simulink model "c71_car0_template"  (R2025b)
settings: Solver=FixedStepDiscrete  StartTime=0.0  StopTime=inf  FixedStep=P_dt  RelTol=1e-3
InitFcn:
  | rosenv;
  | s06_data;
model workspace (MAT data in the model file):
  SL_ROS_VariableLengthArrays_MaxSizes.CommonInfo.ArrayTruncateAction = 'DoNothing'
  SL_ROS_VariableLengthArrays_MaxSizes.MsgTypeMap = containers.Map
  SL_ROS_VariableLengthArrays_MaxSizes.MsgTypeMap.serialization.keys = {'mbmadmsgs/CarObsList', 'mbmadmsgs/CarOutputsExtList', 'mbmadmsgs/DriveManeuver', 'mbsafemsgs/CheckpointSequence'}
  SL_ROS_VariableLengthArrays_MaxSizes.MsgTypeMap.serialization.values{1}.PropertyName = 'list'
  SL_ROS_VariableLengthArrays_MaxSizes.MsgTypeMap.serialization.values{1}.DataType = 'mbmadmsgs/CarObs'
  SL_ROS_VariableLengthArrays_MaxSizes.MsgTypeMap.serialization.values{1}.MaxLength = 4
  SL_ROS_VariableLengthArrays_MaxSizes.MsgTypeMap.serialization.values{2}.PropertyName = 'list'
  SL_ROS_VariableLengthArrays_MaxSizes.MsgTypeMap.serialization.values{2}.DataType = 'mbmadmsgs/CarOutputsExt'
  SL_ROS_VariableLengthArrays_MaxSizes.MsgTypeMap.serialization.values{2}.MaxLength = 2
  SL_ROS_VariableLengthArrays_MaxSizes.MsgTypeMap.serialization.values{3}(1).PropertyName = 'breaks'
  SL_ROS_VariableLengthArrays_MaxSizes.MsgTypeMap.serialization.values{3}(1).DataType = 'single'
  SL_ROS_VariableLengthArrays_MaxSizes.MsgTypeMap.serialization.values{3}(1).MaxLength = 200
  SL_ROS_VariableLengthArrays_MaxSizes.MsgTypeMap.serialization.values{3}(2).PropertyName = 's1'
  SL_ROS_VariableLengthArrays_MaxSizes.MsgTypeMap.serialization.values{3}(2).DataType = 'single'
  SL_ROS_VariableLengthArrays_MaxSizes.MsgTypeMap.serialization.values{3}(2).MaxLength = 200
  SL_ROS_VariableLengthArrays_MaxSizes.MsgTypeMap.serialization.values{3}(3).PropertyName = 's2'
  SL_ROS_VariableLengthArrays_MaxSizes.MsgTypeMap.serialization.values{3}(3).DataType = 'single'
  SL_ROS_VariableLengthArrays_MaxSizes.MsgTypeMap.serialization.values{3}(3).MaxLength = 200
  SL_ROS_VariableLengthArrays_MaxSizes.MsgTypeMap.serialization.values{3}(4).PropertyName = 'segments'
  SL_ROS_VariableLengthArrays_MaxSizes.MsgTypeMap.serialization.values{3}(4).DataType = 'uint32'
  SL_ROS_VariableLengthArrays_MaxSizes.MsgTypeMap.serialization.values{3}(4).MaxLength = 200
  SL_ROS_VariableLengthArrays_MaxSizes.MsgTypeMap.serialization.values{3}(5).PropertyName = 'spline_coefs1'
  SL_ROS_VariableLengthArrays_MaxSizes.MsgTypeMap.serialization.values{3}(5).DataType = 'single'
  SL_ROS_VariableLengthArrays_MaxSizes.MsgTypeMap.serialization.values{3}(5).MaxLength = 800
  SL_ROS_VariableLengthArrays_MaxSizes.MsgTypeMap.serialization.values{3}(6).PropertyName = 'spline_coefs2'
  SL_ROS_VariableLengthArrays_MaxSizes.MsgTypeMap.serialization.values{3}(6).DataType = 'single'
  SL_ROS_VariableLengthArrays_MaxSizes.MsgTypeMap.serialization.values{3}(6).MaxLength = 800
  SL_ROS_VariableLengthArrays_MaxSizes.MsgTypeMap.serialization.values{4}.PropertyName = 'cpseq'
  SL_ROS_VariableLengthArrays_MaxSizes.MsgTypeMap.serialization.values{4}.DataType = 'mbsafemsgs/Checkpoint'
  SL_ROS_VariableLengthArrays_MaxSizes.MsgTypeMap.serialization.values{4}.MaxLength = 23
  SL_ROS_VariableLengthArrays_MaxSizes.MsgTypeMap.serialization.uniformity = 0
  SL_ROS_VariableLengthArrays_MaxSizes.MsgTypeMap.serialization.keyType = 'char'
  SL_ROS_VariableLengthArrays_MaxSizes.MsgTypeMap.serialization.valueType = 'any'
values from neighbouring files (symbols this model uses):
  P_display_dt = 50e-3    (= 0.05)    [s06_data.m]
  P_dt = 25e-3    (= 0.025)    [s06_data.m]
  P_p_delta_max = 21.58/180*pi    (= 0.37664205258)    [d01_data.m]    (also in d71_data.m = 0.383972435439)
  P_p_deltan_max = 1    [d01_data.m]    (also in d71_data.m = 0.93)
  P_p_deltan_min = -P_p_deltan_max    (= -1)    [d01_data.m]    (also in d71_data.m = -0.93)
  P_p_k = 2.51    [d01_data.m]    (also in d71_data.m = 3.4)
  P_p_l = abs(P_p_frontaxle_1 + P_p_rearaxle_1)    [d01_data.m]    (also in d71_data.m = 0.0325)
  P_p_T = 316e-3    (= 0.316)    [d01_data.m]    (also in d71_data.m = 0.12)
  P_p_Tsteer = 0.3    [d01_data.m]
  P_p_Tt = P_p_uTt + P_p_output_Tt    (= 0.11)    [d01_data.m]    (also in d71_data.m = 0.1)
  P_p_un_max = 1    [d01_data.m]    (also in d71_data.m = 0.2)
  P_p_vRef = 0.2    [baseline_lqr_script.m]    (also in d71_data.m = 0.15)
undefined symbols (not defined in the file or in its folder): carid, CarInputsCmdForward, CarInputsCmdHalt, cmd, cpseq, P_cpseq, P_p_tuneKI, P_p_tuneKP, P_p_un_table, P_p_uref, P_p_vss_table, pedals, steering
libraries: ros2lib x5, mbrt_lib_level1 x2, vrlib x1, eeGeneralControl x1
settings Model: Creator=frank  LastModifiedBy=jty
settings OptimizationCC: EnhancedBackFolding=on  PassReuseOutputArgsAs=Individual arguments  ZeroExternalMemoryAtStartup=off  ZeroInternalMemoryAtStartup=off  MaxStackSize=64  OptimizeBlockOrder=speed  DifferentSizesBufferReuse=on  OptimizationCustomize=off  EfficientTunableParamExpr=on
settings DebuggingCC: ParameterTunabilityLossMsg=error  UnconnectedInputMsg=warning  UnconnectedOutputMsg=warning  UnconnectedLineMsg=warning  BusObjectLabelMismatch=error
settings HardwareCC: ProdBitPerLong=64.0  ProdHWDeviceType=Intel->x86-64 (Linux 64)
settings ModelReferenceCC: EnableRefExpFcnMdlSchedulingChecks=on
settings SFSimCC: MATLABDynamicMemAlloc=off
settings RTWCC: SystemTargetFile=ert.tlc  HardwareBoard=Robot Operating System 2 (ROS 2)  GenCodeOnly=on  TemplateMakefile=ert_default_tmf  GenerateReport=on  Toolchain=Colcon Tools  BuildConfiguration=Faster Runs  IncludeHyperlinkInReport=on  TargetLang=C++  GenerateTraceInfo=on  GPUComputeCapability=3.5  DLArmComputeVersion=19.05  Description=Embedded Coder
settings CodeAppCC: ForceParamTrailComments=on  IgnoreCustomStorageClasses=off  OperatorAnnotations=on  SimulinkDataObjDesc=on  SFDataObjDesc=on  InsertBlockDesc=on
settings ERTTargetCC: ExtModeTransport=2.0  ExtModeStaticAlloc=on  ExtModeAutomaticAllocSize=off  ExtModeMexFile=ext_xcp  ExtModeIntrfLevel=Level2 - Open  InlinedParameterPlacement=Hierarchical  RootIOFormat=Structure reference  DynamicArrayContainerType=coder::array  CodeInterfacePackaging=C++ class  SubcomponentCodeInterfacePackaging=C++ class  SupportNonInlinedSFcns=on  SupportVariableSizeSignals=on

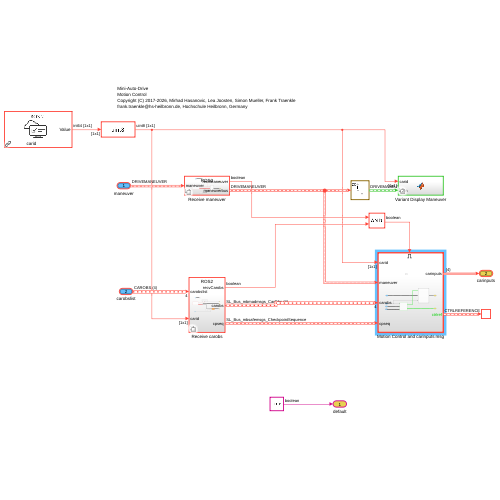
[thumbnail: Simulink's stored preview of the top-level diagram]
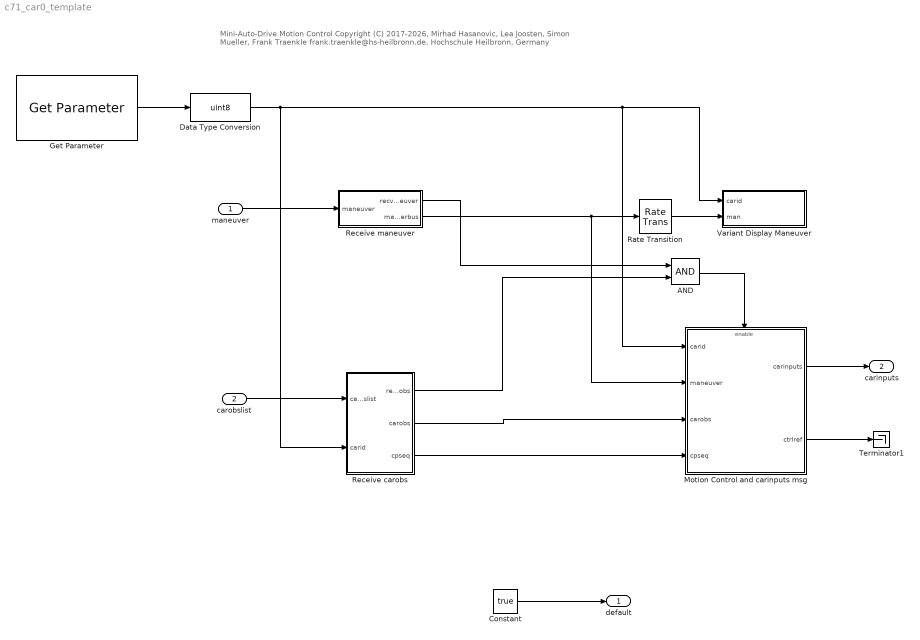
== system c71_car0_template ==
  note: Mini-Auto-Drive
      | Motion Control
      | Copyright (C) 2017-2026, Mirhad Hasanovic, Lea Joosten, Simon Mueller, Frank Traenkle
      | frank.traenkle@hs-heilbronn.de, Hochschule Heilbronn, Germany
  maneuver : Inport  OutDataTypeStr=Bus: DRIVEMANEUVER  BusOutputAsStruct=on
  carobslist : Inport  Port=2  OutDataTypeStr=Bus: CAROBS  PortDimensions=P_car_cnt  BusOutputAsStruct=on
  AND : Logic  AllPortsSameDT=off  OutDataTypeStr=boolean
  Constant : Constant  Value=true
  Data Type Conversion : DataTypeConversion  OutDataTypeStr=uint8  SaturateOnIntegerOverflow=off  RndMeth=Floor
  Get Parameter : ros2lib/Get Parameter  ParameterName=carid  ParameterType=int64  ParameterMaxArrayLength=16  ParameterInitialValue=0  SampleTime=-1  ModelName=c71_car0_template  BlockId=ParamGet_c71_car0_template_2057
  Motion Control and carinputs msg : Subsystem
  Rate Transition : RateTransition
  Receive carobs : Subsystem  Variant=on
  Receive maneuver : Subsystem  Variant=on
  Terminator1 : Terminator
  Variant Display Maneuver : Subsystem  Variant=on  VariantControlMode=sim codegen switching
  default : Outport  BusOutputAsStruct=on
  carinputs : Outport  Port=2  OutDataTypeStr=Bus: CARINPUTS  BusOutputAsStruct=on
  wires:
  Receive maneuver/1(recvManeuver) -> AND/1
  Motion Control and carinputs msg/1(carinputs) -> carinputs/1
  Receive maneuver/2(maneuverbus) -> Motion Control and carinputs msg/2(maneuver), Rate Transition/1
  Motion Control and carinputs msg/2(ctrlref) -> Terminator1/1
  Rate Transition/1 -> Variant Display Maneuver/2(man)
  maneuver/1 -> Receive maneuver/1(maneuver)
  Receive carobs/2(carobs) -> Motion Control and carinputs msg/3(carobs)
  Data Type Conversion/1 -> Receive carobs/2(carid), Motion Control and carinputs msg/1(carid), Variant Display Maneuver/1(carid)
  Receive carobs/3(cpseq) -> Motion Control and carinputs msg/4(cpseq)
  AND/1 -> Motion Control and carinputs msg/Enable
  Receive carobs/1(recvCarobs) -> AND/2
  carobslist/1 -> Receive carobs/1(carobslist)
  Constant/1 -> default/1
  Get Parameter/1 -> Data Type Conversion/1

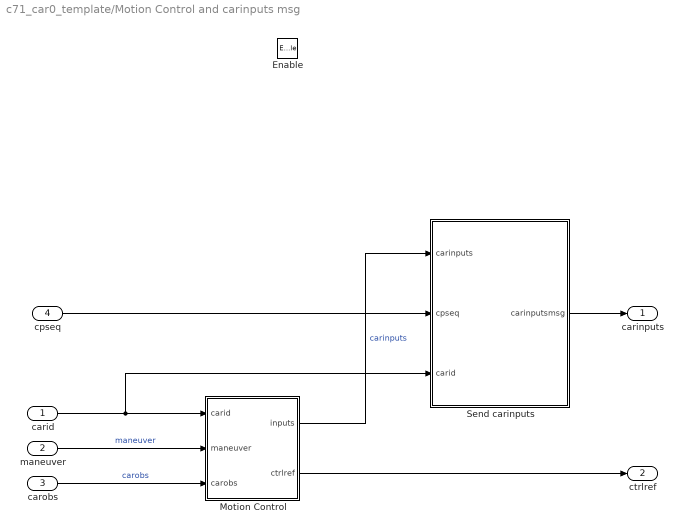
== system c71_car0_template/Motion Control and carinputs msg ==
  carid : Inport
  maneuver : Inport  Port=2
  carobs : Inport  Port=3
  cpseq : Inport  Port=4
  Enable : EnablePort
  Motion Control : Subsystem  TreatAsAtomicUnit=on  SystemSampleTime=P_dt
  Send carinputs : Subsystem  Variant=on
  carinputs : Outport
  ctrlref : Outport  Port=2
  wires:
  Send carinputs/1(carinputsmsg) -> carinputs/1
  carid/1 -> Motion Control/1(carid), Send carinputs/3(carid)
  cpseq/1 -> Send carinputs/2(cpseq)
  Motion Control/1(inputs) -> Send carinputs/1(carinputs)  "carinputs"
  Motion Control/2(ctrlref) -> ctrlref/1
  carobs/1 -> Motion Control/3(carobs)  "carobs"
  maneuver/1 -> Motion Control/2(maneuver)  "maneuver"

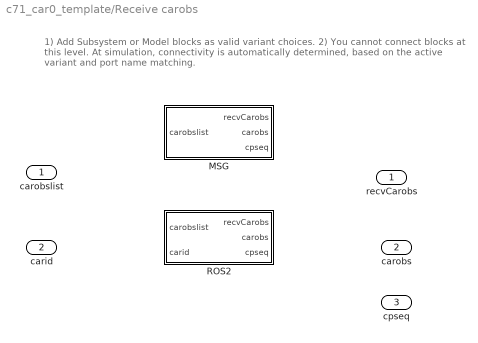
== system c71_car0_template/Receive carobs ==
  note: 1) Add Subsystem or Model blocks as valid variant choices.
      | 2) You cannot connect blocks at this level. At simulation, connectivity is automatically
      | determined, based on the active variant and port name matching.
  carobslist : Inport
  carid : Inport  Port=2
  MSG : Subsystem  VariantControl=VariantCom == VARIANT_COM_TYPE.MSG
  ROS2 : Subsystem  VariantControl=VariantCom == VARIANT_COM_TYPE.ROS2
  recvCarobs : Outport
  carobs : Outport  Port=2
  cpseq : Outport  Port=3

== system c71_car0_template/Receive maneuver ==
  note: 1) Add Subsystem or Model blocks as valid variant choices.
      | 2) You cannot connect blocks at this level. At simulation, connectivity is automatically
      | determined, based on the active variant and port name matching.
  maneuver : Inport
  MSG : Subsystem  VariantControl=VariantCom == VARIANT_COM_TYPE.MSG
  ROS2 : Subsystem  VariantControl=VariantCom == VARIANT_COM_TYPE.ROS2
  recvManeuver : Outport
  maneuverbus : Outport  Port=2

== system c71_car0_template/Variant Display Maneuver ==
  note: 1) Add Subsystem or Model blocks as valid variant choices.
      | 2) You cannot connect blocks at this level. At simulation, connectivity is automatically
      | determined, based on the active variant and port name matching.
  carid : Inport
  man : Inport  Port=2
  DisplayManeuver : MATLAB Function  TreatAsAtomicUnit=on  SystemSampleTime=P_display_dt  VariantControl=(sim)
  None : Subsystem  VariantControl=(codegen)

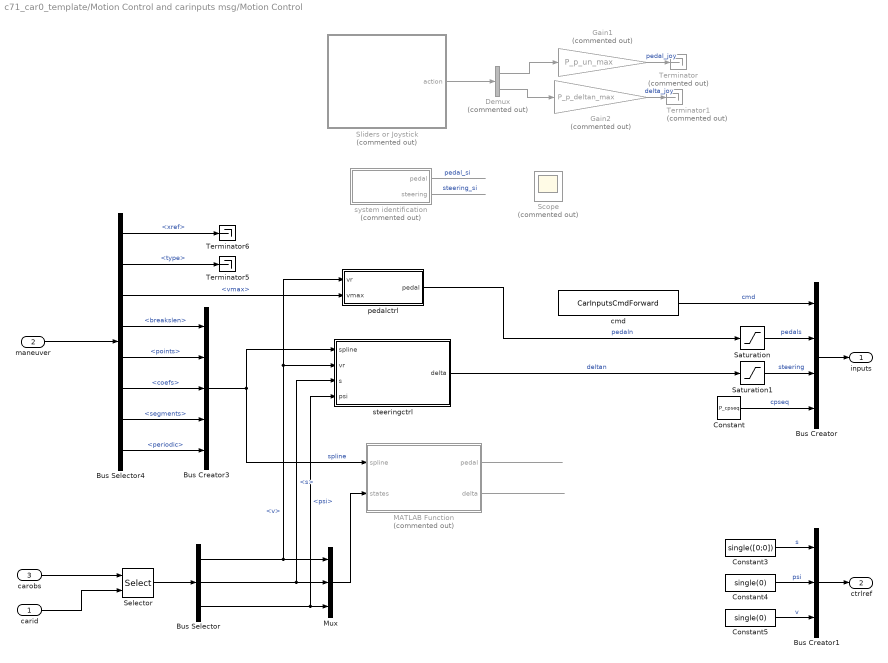
== system c71_car0_template/Motion Control and carinputs msg/Motion Control ==
  carid : Inport
  maneuver : Inport  Port=2
  carobs : Inport  Port=3
  Bus Creator : BusCreator  Inputs=4  OutDataTypeStr=Bus: CARINPUTS  NonVirtualBus=on
  Bus Creator1 : BusCreator  Inputs=3  OutDataTypeStr=Bus: CTRLREFERENCE  NonVirtualBus=on
  Bus Creator3 : BusCreator  Inputs=5  OutDataTypeStr=Bus: SPLINE
  Bus Selector : BusSelector  OutputSignals=v,s,psi
  Bus Selector4 : BusSelector  OutputSignals=xref,type,vmax,breakslen,points,coefs,segments,periodic
  Constant : Constant  Value=P_cpseq  OutDataTypeStr=Bus: CHECKPOINTSEQUENCEMSG
  Constant3 : Constant  Value=single([0;0])
  Constant4 : Constant  Value=single(0)
  Constant5 : Constant  Value=single(0)
  Demux : Demux  Commented=on  Outputs=2
  Gain1 : Gain  Commented=on  Gain=P_p_un_max
  Gain2 : Gain  Commented=on  Gain=P_p_deltan_max
  MATLAB Function : MATLAB Function  Commented=on  TreatAsAtomicUnit=on
  Mux : Mux  Inputs=3
  Saturation : Saturate  UpperLimit=P_p_un_max  LowerLimit=0.03
  Saturation1 : Saturate  UpperLimit=P_p_deltan_max  LowerLimit=P_p_deltan_min
  Scope : Scope  Commented=on  NumInputPorts=2
      settings: ActiveDisplayYMinimum=-0.15337172032176821  ActiveDisplayYMaximum=0.22733787891864379
  Selector : Selector  IndexMode=Zero-based  InputPortWidth=P_car_cnt  IndexOptions=Index vector (port)  Indices=0  OutputSizes=1
  Sliders or Joystick : Subsystem  Commented=on  Variant=on  VariantControlMode=label  LabelModeActiveChoice=true
  Terminator : Terminator  Commented=on
  Terminator1 : Terminator  Commented=on
  Terminator5 : Terminator
  Terminator6 : Terminator
  cmd : Constant  Value=CarInputsCmdForward
  pedalctrl : Subsystem
  steeringctrl : Subsystem
  system identification : Subsystem  Commented=on
  inputs : Outport  VectorParamsAs1DForOutWhenUnconnected=off
  ctrlref : Outport  Port=2  VectorParamsAs1DForOutWhenUnconnected=off
  wires:
  Constant5/1 -> Bus Creator1/3  "v"
  Constant3/1 -> Bus Creator1/1  "s"
  Constant4/1 -> Bus Creator1/2  "psi"
  Bus Creator1/1 -> ctrlref/1
  Constant/1 -> Bus Creator/4  "cpseq"
  Demux/2 -> Gain2/1
  Demux/1 -> Gain1/1
  Sliders or Joystick/1(action) -> Demux/1
  Bus Creator/1 -> inputs/1
  Saturation/1 -> Bus Creator/2  "pedals"
  Saturation1/1 -> Bus Creator/3  "steering"
  cmd/1 -> Bus Creator/1  "cmd"
  Gain2/1 -> Terminator1/1  "delta_joy"
  Gain1/1 -> Terminator/1  "pedal_joy"
  Bus Selector/2 -> steeringctrl/3(s), Mux/2  "<s>"
  carobs/1 -> Selector/1
  Bus Selector/1 -> pedalctrl/1(vr), steeringctrl/2(vr), Mux/1  "<v>"
  Bus Selector/3 -> steeringctrl/4(psi), Mux/3  "<psi>"
  Selector/1 -> Bus Selector/1
  carid/1 -> Selector/2
  Bus Selector4/7 -> Bus Creator3/4  "<segments>"
  Bus Selector4/2 -> Terminator5/1  "<type>"
  maneuver/1 -> Bus Selector4/1
  Bus Selector4/3 -> pedalctrl/2(vmax)  "<vmax>"
  Bus Selector4/8 -> Bus Creator3/5  "<periodic>"
  Bus Creator3/1 -> MATLAB Function/1(spline), steeringctrl/1(spline)  "spline"
  Bus Selector4/1 -> Terminator6/1  "<xref>"
  Bus Selector4/6 -> Bus Creator3/3  "<coefs>"
  Bus Selector4/5 -> Bus Creator3/2  "<points>"
  Bus Selector4/4 -> Bus Creator3/1  "<breakslen>"
  pedalctrl/1(pedal) -> Saturation/1  "pedaln"
  steeringctrl/1(delta) -> Saturation1/1  "deltan"
  system identification/1(pedal) -> ?  "pedal_si"
  system identification/2(steering) -> ?  "steering_si"
  Mux/1 -> MATLAB Function/2(states)
  MATLAB Function/1(pedal) -> ?
  MATLAB Function/2(delta) -> ?

== system c71_car0_template/Motion Control and carinputs msg/Send carinputs ==
  note: 1) Add Subsystem or Model blocks as valid variant choices.
      | 2) You cannot connect blocks at this level. At simulation, connectivity is automatically
      | determined, based on the active variant and port name matching.
  carinputs : Inport
  cpseq : Inport  Port=2
  carid : Inport  Port=3
  MSG : Subsystem  VariantControl=VariantCom == VARIANT_COM_TYPE.MSG
  ROS2 : Subsystem  VariantControl=VariantCom == VARIANT_COM_TYPE.ROS2
  carinputsmsg : Outport

== system c71_car0_template/Receive carobs/MSG ==
  carobslist : Inport  OutDataTypeStr=Bus: CAROBS  BusOutputAsStruct=on
  Constant : Constant  Value=P_cpseq  OutDataTypeStr=Bus: CHECKPOINTSEQUENCEMSG
  Message Receive1 : Receive  InputPortMessageModes=m  UseInternalQueue=off  QueueLength=1  ShowQueueStatus=on
      settings: OutputPortMap=o0,o1
  recvCarobs : Outport
  carobs : Outport  Port=2
  cpseq : Outport  Port=3
  wires:
  Message Receive1/2 -> carobs/1
  Message Receive1/1 -> recvCarobs/1
  Constant/1 -> cpseq/1
  carobslist/1 -> Message Receive1/1

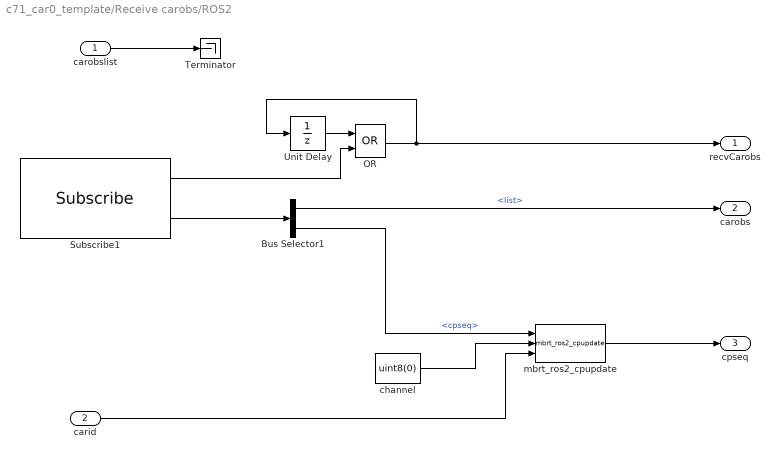
== system c71_car0_template/Receive carobs/ROS2 ==
  carobslist : Inport  OutDataTypeStr=Bus: CAROBS  BusOutputAsStruct=on
  carid : Inport  Port=2
  Bus Selector1 : BusSelector  OutputSignals=list,cpseq
  OR : Logic  Operator=OR  AllPortsSameDT=off  OutDataTypeStr=boolean
  Subscribe1 : ros2lib/Subscribe  topicSource=Specify your own  topic=/mad/locate/carobs  messageType=mbmadmsgs/CarObsList  sampleTime=-1  QOSHistory=Keep last  QOSDepth=1  QOSReliability=Best effort  QOSDurability=Volatile  QOSDeadline=Inf  QOSLifespan=Inf  QOSLiveliness=Automatic  QOSLeaseDuration=Inf  QOSAvoidROSNamespaceConventions=off
  Terminator : Terminator
  Unit Delay : UnitDelay  InitialCondition=false  SampleTime=-1  HasFrameUpgradeWarning=on
  channel : Constant  Value=uint8(0)
  mbrt_ros2_cpupdate : mbrt_lib_level1/mbrt_ros2_cpupdate  P_cur_cpid=P_cpid_CtrlStart
  recvCarobs : Outport
  carobs : Outport  Port=2
  cpseq : Outport  Port=3
  wires:
  Bus Selector1/2 -> mbrt_ros2_cpupdate/1  "<cpseq>"
  OR/1 -> recvCarobs/1, Unit Delay/1
  Subscribe1/1 -> OR/2
  Bus Selector1/1 -> carobs/1  "<list>"
  channel/1 -> mbrt_ros2_cpupdate/2
  mbrt_ros2_cpupdate/1 -> cpseq/1
  carobslist/1 -> Terminator/1
  Subscribe1/2 -> Bus Selector1/1
  Unit Delay/1 -> OR/1
  carid/1 -> mbrt_ros2_cpupdate/3

== system c71_car0_template/Receive maneuver/MSG ==
  maneuver : Inport  OutDataTypeStr=Bus: DRIVEMANEUVER  BusOutputAsStruct=on
  Message Receive : Receive  InputPortMessageModes=m  UseInternalQueue=off  QueueLength=1  ShowQueueStatus=on
      settings: OutputPortMap=o0,o1
  recvManeuver : Outport
  maneuverbus : Outport  Port=2
  wires:
  Message Receive/2 -> maneuverbus/1
  Message Receive/1 -> recvManeuver/1
  maneuver/1 -> Message Receive/1

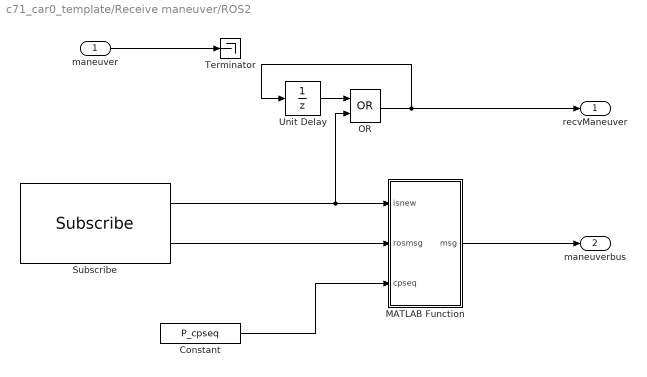
== system c71_car0_template/Receive maneuver/ROS2 ==
  maneuver : Inport  OutDataTypeStr=Bus: DRIVEMANEUVER  BusOutputAsStruct=on
  Constant : Constant  Value=P_cpseq  OutDataTypeStr=Bus: CHECKPOINTSEQUENCEMSG
  MATLAB Function : MATLAB Function  TreatAsAtomicUnit=on
  OR : Logic  Operator=OR  AllPortsSameDT=off  OutDataTypeStr=boolean
  Subscribe : ros2lib/Subscribe  topicSource=Select from ROS network  topic=/mad/car0/maneuver  messageType=mbmadmsgs/DriveManeuver  sampleTime=-1  QOSHistory=Keep last  QOSDepth=1  QOSReliability=Best effort  QOSDurability=Volatile  QOSDeadline=Inf  QOSLifespan=Inf  QOSLiveliness=Automatic  QOSLeaseDuration=Inf  QOSAvoidROSNamespaceConventions=off
  Terminator : Terminator
  Unit Delay : UnitDelay  InitialCondition=false  SampleTime=-1  HasFrameUpgradeWarning=on
  recvManeuver : Outport
  maneuverbus : Outport  Port=2
  wires:
  MATLAB Function/1(msg) -> maneuverbus/1
  maneuver/1 -> Terminator/1
  Subscribe/1 -> OR/2, MATLAB Function/1(isnew)
  Subscribe/2 -> MATLAB Function/2(rosmsg)
  Constant/1 -> MATLAB Function/3(cpseq)
  OR/1 -> recvManeuver/1, Unit Delay/1
  Unit Delay/1 -> OR/1

== system c71_car0_template/Variant Display Maneuver/None ==
  carid : Inport
  man : Inport  Port=2

== system c71_car0_template/Motion Control and carinputs msg/Motion Control/Sliders or Joystick ==
  note: 1) Add Subsystem or Model blocks as valid variant choices.
      | 2) You cannot connect blocks at this level. At simulation, connectivity is automatically
      | determined, based on the active variant and port name matching.
  Joystick : Subsystem  VariantControl=false
  Sliders : Subsystem  VariantControl=true
  action : Outport

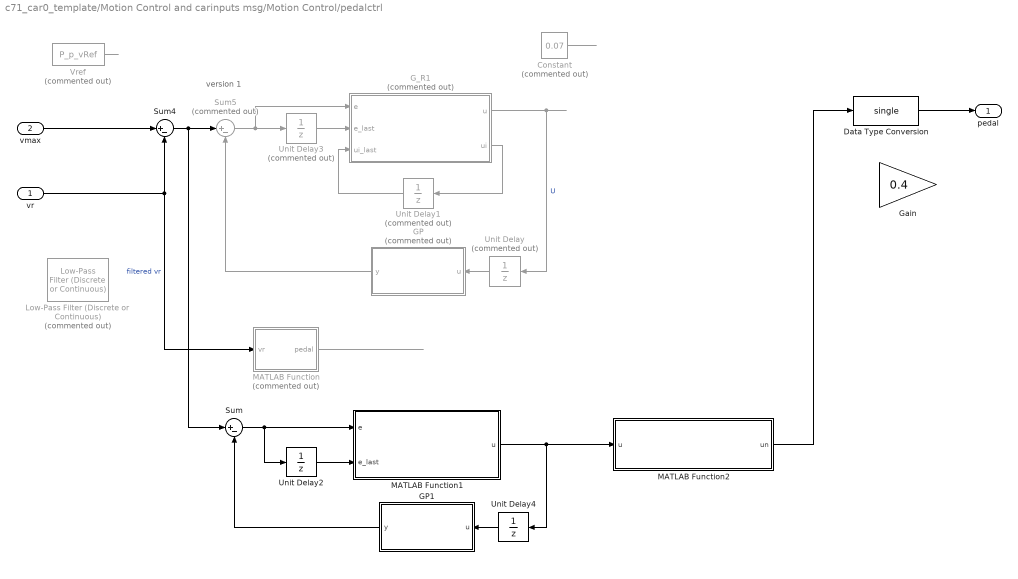
== system c71_car0_template/Motion Control and carinputs msg/Motion Control/pedalctrl ==
  note: version 1
  vr : Inport
  vmax : Inport  Port=2
  Constant : Constant  Commented=on  Value=0.07
  Data Type Conversion : DataTypeConversion  OutDataTypeStr=single  SaturateOnIntegerOverflow=off  RndMeth=Floor
  GP : MATLAB Function  Commented=on  TreatAsAtomicUnit=on
  GP1 : MATLAB Function  TreatAsAtomicUnit=on
  G_R1 : MATLAB Function  Commented=on  TreatAsAtomicUnit=on
  Gain : Gain  Gain=0.4
  Low-Pass Filter (Discrete or Continuous) : eeGeneralControl/Low-Pass Filter (Discrete or Continuous)  Commented=on  K=1  T=0.05  B=inf  A=-inf  init_option=Inherited from block input  x0=0  Ts=-1
  MATLAB Function : MATLAB Function  Commented=on  TreatAsAtomicUnit=on
  MATLAB Function1 : MATLAB Function  TreatAsAtomicUnit=on
  MATLAB Function2 : MATLAB Function  TreatAsAtomicUnit=on
  Sum : Sum  Inputs=|+-
  Sum4 : Sum  Inputs=|+-
  Sum5 : Sum  Commented=on  Inputs=|+-
  Unit Delay : UnitDelay  Commented=on  SampleTime=-1
  Unit Delay1 : UnitDelay  Commented=on  SampleTime=-1  HasFrameUpgradeWarning=on
  Unit Delay2 : UnitDelay  SampleTime=-1  HasFrameUpgradeWarning=on
  Unit Delay3 : UnitDelay  Commented=on  SampleTime=-1  HasFrameUpgradeWarning=on
  Unit Delay4 : UnitDelay  SampleTime=-1  HasFrameUpgradeWarning=on
  Vref : Constant  Commented=on  Value=P_p_vRef
  pedal : Outport
  wires:
  MATLAB Function/1(pedal) -> ?
  Unit Delay1/1 -> G_R1/3(ui_last)
  Sum4/1 -> Sum/1, Sum5/1
  Unit Delay3/1 -> G_R1/2(e_last)
  Unit Delay/1 -> GP/1(u)
  Sum5/1 -> G_R1/1(e), Unit Delay3/1
  GP/1(y) -> Sum5/2
  G_R1/2(ui) -> Unit Delay1/1
  G_R1/1(u) -> Unit Delay/1  "U"
  Vref/1 -> ?
  Constant/1 -> ?
  vr/1 -> MATLAB Function/1(vr), Sum4/2  "filtered vr"
  vmax/1 -> Sum4/1
  Data Type Conversion/1 -> pedal/1
  Unit Delay2/1 -> MATLAB Function1/2(e_last)
  MATLAB Function1/1(u) -> MATLAB Function2/1(u), Unit Delay4/1
  Unit Delay4/1 -> GP1/1(u)
  Sum/1 -> Unit Delay2/1, MATLAB Function1/1(e)
  GP1/1(y) -> Sum/2
  MATLAB Function2/1(un) -> Data Type Conversion/1

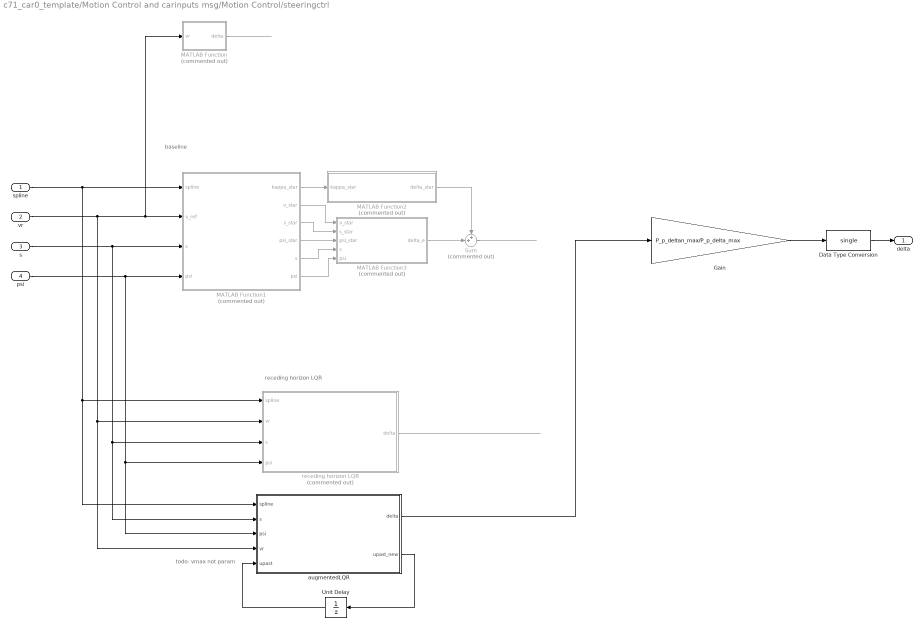
== system c71_car0_template/Motion Control and carinputs msg/Motion Control/steeringctrl ==
  note: todo: vmax not param
  note: receding horizon LQR
  note: baseline
  spline : Inport
  vr : Inport  Port=2
  s : Inport  Port=3
  psi : Inport  Port=4
  Data Type Conversion : DataTypeConversion  OutDataTypeStr=single  SaturateOnIntegerOverflow=off  RndMeth=Floor
  Gain : Gain  Gain=P_p_deltan_max/P_p_delta_max
  MATLAB Function : MATLAB Function  Commented=on  TreatAsAtomicUnit=on
  MATLAB Function1 : MATLAB Function  Commented=on  TreatAsAtomicUnit=on
  MATLAB Function2 : MATLAB Function  Commented=on  TreatAsAtomicUnit=on
  MATLAB Function3 : MATLAB Function  Commented=on  TreatAsAtomicUnit=on
  Sum : Sum  Commented=on  Inputs=++|
  Unit Delay : UnitDelay  InitialCondition=[0;0;0;0]  SampleTime=-1  HasFrameUpgradeWarning=on
  augmentedLQR : MATLAB Function  TreatAsAtomicUnit=on
  receding horizon LQR : MATLAB Function  Commented=on  TreatAsAtomicUnit=on
  delta : Outport
  wires:
  vr/1 -> augmentedLQR/4(vr), receding horizon LQR/2(vr), MATLAB Function/1(vr), MATLAB Function1/2(v_ref)
  MATLAB Function/1(delta) -> ?
  Data Type Conversion/1 -> delta/1
  spline/1 -> augmentedLQR/1(spline), receding horizon LQR/1(spline), MATLAB Function1/1(spline)
  s/1 -> augmentedLQR/2(s), receding horizon LQR/3(s), MATLAB Function1/3("s ")
  MATLAB Function1/1(kappa_star) -> MATLAB Function2/1(kappa_star)
  MATLAB Function1/2(v_star) -> MATLAB Function3/1(v_star)
  MATLAB Function1/3(s_star) -> MATLAB Function3/2(s_star)
  MATLAB Function1/4(psi_star) -> MATLAB Function3/3(psi_star)
  psi/1 -> MATLAB Function1/4("psi "), augmentedLQR/3(psi), receding horizon LQR/4(psi)
  MATLAB Function1/5(s) -> MATLAB Function3/4(s)
  MATLAB Function1/6(psi) -> MATLAB Function3/5(psi)
  MATLAB Function3/1(delta_e) -> Sum/2
  MATLAB Function2/1(delta_star) -> Sum/1
  Sum/1 -> ?
  Gain/1 -> Data Type Conversion/1
  receding horizon LQR/1(delta) -> ?
  augmentedLQR/2(upast_new) -> Unit Delay/1
  Unit Delay/1 -> augmentedLQR/5(upast)
  augmentedLQR/1(delta) -> Gain/1

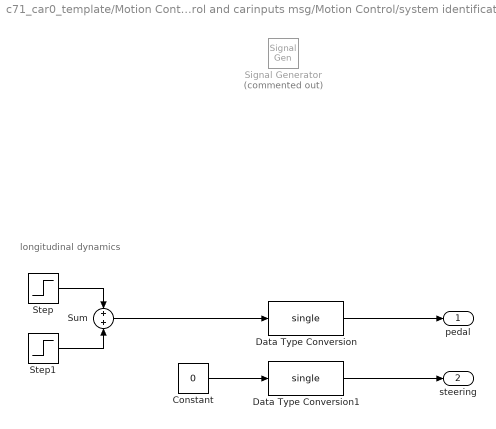
== system c71_car0_template/Motion Control and carinputs msg/Motion Control/system identification ==
  note: longitudinal dynamics
  Constant : Constant  Value=0
  Data Type Conversion : DataTypeConversion  OutDataTypeStr=single  SaturateOnIntegerOverflow=off  RndMeth=Floor
  Data Type Conversion1 : DataTypeConversion  OutDataTypeStr=single  SaturateOnIntegerOverflow=off  RndMeth=Floor
  Signal Generator : SignalGenerator  Commented=on  Units=rad/sec
  Step : Step  Time=5  After=P_p_uref  SampleTime=P_dt
  Step1 : Step  Time=5.75  After=-P_p_uref  SampleTime=P_dt
  Sum : Sum  Inputs=+|+
  pedal : Outport
  steering : Outport  Port=2
  wires:
  Step/1 -> Sum/1
  Step1/1 -> Sum/2
  Sum/1 -> Data Type Conversion/1
  Constant/1 -> Data Type Conversion1/1
  Data Type Conversion/1 -> pedal/1
  Data Type Conversion1/1 -> steering/1

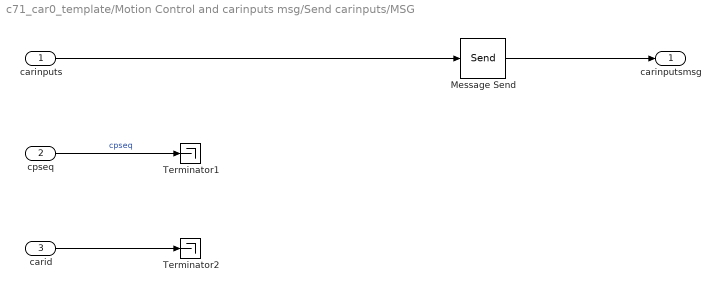
== system c71_car0_template/Motion Control and carinputs msg/Send carinputs/MSG ==
  carinputs : Inport
  cpseq : Inport  Port=2
  carid : Inport  Port=3
  Message Send : Send  OutputPortMessageModes=m
  Terminator1 : Terminator
  Terminator2 : Terminator
  carinputsmsg : Outport
  wires:
  Message Send/1 -> carinputsmsg/1
  carid/1 -> Terminator2/1
  carinputs/1 -> Message Send/1
  cpseq/1 -> Terminator1/1  "cpseq"

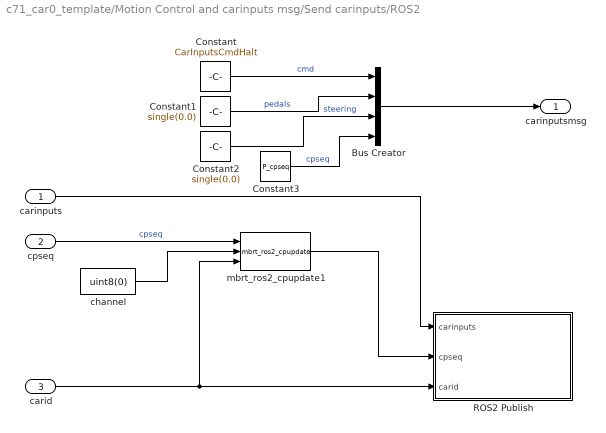
== system c71_car0_template/Motion Control and carinputs msg/Send carinputs/ROS2 ==
  carinputs : Inport
  cpseq : Inport  Port=2
  carid : Inport  Port=3
  Bus Creator : BusCreator  Inputs=4  OutDataTypeStr=Bus: CARINPUTS
  Constant : Constant  Value=CarInputsCmdHalt  SampleTime=-1
  Constant1 : Constant  Value=single(0.0)  SampleTime=-1
  Constant2 : Constant  Value=single(0.0)  SampleTime=-1
  Constant3 : Constant  Value=P_cpseq  OutDataTypeStr=Bus: CHECKPOINTSEQUENCEMSG  SampleTime=-1
  ROS2 Publish : Subsystem
  channel : Constant  Value=uint8(0)
  mbrt_ros2_cpupdate1 : mbrt_lib_level1/mbrt_ros2_cpupdate  P_cur_cpid=P_cpid_CtrlPublish
  carinputsmsg : Outport
  wires:
  carinputs/1 -> ROS2 Publish/1(carinputs)
  cpseq/1 -> mbrt_ros2_cpupdate1/1  "cpseq"
  Bus Creator/1 -> carinputsmsg/1
  mbrt_ros2_cpupdate1/1 -> ROS2 Publish/2(cpseq)
  carid/1 -> mbrt_ros2_cpupdate1/3, ROS2 Publish/3(carid)
  channel/1 -> mbrt_ros2_cpupdate1/2
  Constant/1 -> Bus Creator/1  "cmd"
  Constant1/1 -> Bus Creator/2  "pedals"
  Constant2/1 -> Bus Creator/3  "steering"
  Constant3/1 -> Bus Creator/4  "cpseq"

== system c71_car0_template/Motion Control and carinputs msg/Motion Control/Sliders or Joystick/Joystick ==
  Data Type Conversion : DataTypeConversion  OutDataTypeStr=single  SaturateOnIntegerOverflow=off  RndMeth=Floor
  Gain3 : Gain  Gain=-1
  Joystick Input : vrlib/Joystick Input  joyid=1  adjustports=off  forcefeed=off
  Selector1 : Selector  IndexOptions=Index vector (dialog)  Indices=[2 4]  OutputSizes=1
  Terminator : Terminator
  action : Outport
  wires:
  Data Type Conversion/1 -> Selector1/1
  Gain3/1 -> action/1
  Joystick Input/1 -> Data Type Conversion/1
  Selector1/1 -> Gain3/1
  Joystick Input/2 -> Terminator/1

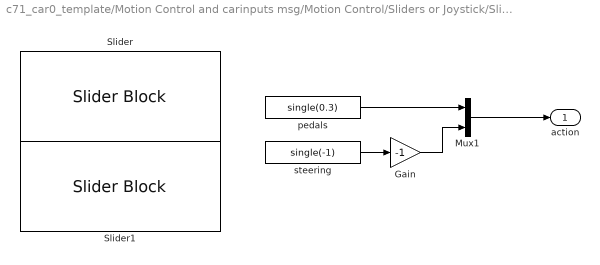
== system c71_car0_template/Motion Control and carinputs msg/Motion Control/Sliders or Joystick/Sliders ==
  Gain : Gain  Gain=-1
  Mux1 : Mux  Inputs=2
  Slider : SliderBlock  ScaleMin=-1  ScaleMax=1
  Slider1 : SliderBlock  ScaleMin=-1  ScaleMax=1
  pedals : Constant  Value=single(0.3)  SampleTime=Inf
  steering : Constant  Value=single(-1)
  action : Outport
  wires:
  pedals/1 -> Mux1/1
  Gain/1 -> Mux1/2
  Mux1/1 -> action/1
  steering/1 -> Gain/1

== system c71_car0_template/Motion Control and carinputs msg/Send carinputs/ROS2/ROS2 Publish ==
  carinputs : Inport
  cpseq : Inport  Port=2
  carid : Inport  Port=3
  Blank Message : ros2lib/Blank Message  messageClass=Message  entityType=mbmadmsgs/CarInputs  messageType=mbmadmsgs/CarInputs  SampleTime=inf
  Bus Assignment : BusAssignment  AssignedSignals=carid,cmd,pedals,steering,cpseq
  Bus Selector : BusSelector  OutputSignals=cmd,pedals,steering
  Publish : ros2lib/Publish  topicSource=Specify your own  topic=/mad/car0/carinputs  messageType=mbmadmsgs/CarInputs  QOSHistory=Keep last  QOSDepth=1  QOSReliability=Best effort  QOSDurability=Volatile  QOSDeadline=Inf  QOSLifespan=Inf  QOSLiveliness=Automatic  QOSLeaseDuration=Inf  QOSAvoidROSNamespaceConventions=off
  wires:
  Bus Selector/2 -> Bus Assignment/4  "<pedals>"
  Bus Selector/1 -> Bus Assignment/3  "<cmd>"
  carid/1 -> Bus Assignment/2
  Bus Selector/3 -> Bus Assignment/5  "<steering>"
  Bus Assignment/1 -> Publish/1
  carinputs/1 -> Bus Selector/1
  Blank Message/1 -> Bus Assignment/1
  cpseq/1 -> Bus Assignment/6

== matlab function c71_car0_template/Motion Control and carinputs msg/Motion Control/pedalctrl/MATLAB Function1 ==
  data: e input; u output; e_last input; P_p_T parameter; P_p_k parameter; P_dt parameter; P_p_tuneKP parameter; P_p_tuneKI parameter
function u = pi_controller(e,e_last,P_p_T, P_p_k, P_dt, P_p_tuneKP, P_p_tuneKI)

   %% from the slides
   Tw = 0.2;
   Kp = P_p_T / (Tw*P_p_k);
   Ki = Kp/P_p_T;
   Ta = P_dt;

   Kp = Kp * P_p_tuneKP;
   Ki = Ki * P_p_tuneKI;

   persistent I_prev
   if isempty(I_prev)
       I_prev = single(0);
   end
   % Tustin integration
   I = I_prev + Ta/2 * (e + e_last);
   % PI controller
   u_unsat = Kp * e + Ki * I;

   % Pedal saturation
   u_min = 0.0;
   u_max = 0.2;
   u = min(max(u_unsat, u_min), u_max);

   % anti-windup
   if (u_unsat > u_max && e > 0) || ...
      (u_unsat < u_min && e < 0)
    
       I = single(I_prev);
    
       % recalculate using frozen integrator
       u_unsat = Kp * e + Ki * I;
       u = min(max(u_unsat, u_min), u_max);
   end

   % save for next sample
   I_prev = I;

   u = single(u);

end

== matlab function c71_car0_template/Motion Control and carinputs msg/Motion Control/pedalctrl/GP1 ==
  data: u input; y output; P_p_Tt parameter; P_dt parameter; P_p_T parameter; P_p_k parameter
function y = SmithPredictor(u, P_p_Tt, P_dt, P_p_T, P_p_k)
    % SMITH PREDICTOR IMPLEMENTATION
    % Calculates the difference between undelayed and delayed plant responses
   
    % delay_steps = round(P_p_Tt / P_dt);
   
    % if delay_steps < 1
    %     delay_steps = 1;
    % end

    delay_steps = 4;
   
    % MEMORY VARIABLES
    persistent y_undelayed_last
    persistent delay_buffer
   
    % INITIALIZATION
    if isempty(y_undelayed_last)
        y_undelayed_last = single(0);
        delay_buffer = zeros(delay_steps, 1, 'single');
    end
   
    % DYNAMIC BUFFER RESIZING
    if length(delay_buffer) ~= delay_steps
        new_buffer = zeros(delay_steps, 1, 'single');
        elements_to_copy = min(length(delay_buffer), delay_steps);
        new_buffer(1:elements_to_copy) = delay_buffer(1:elements_to_copy);
        delay_buffer = new_buffer;
    end
   
    % 1. UNDELAYED PLANT MODEL (Forward Euler)
    y_undelayed = y_undelayed_last + single(P_dt / P_p_T) * (single(P_p_k) * u - y_undelayed_last);
    % can try the exact
   
    % 2. DELAYED PLANT MODEL
    y_delayed = delay_buffer(end);
   
    % 3. BUFFER UPDATE
    if length(delay_buffer) > 1
        delay_buffer(2:end) = delay_buffer(1:end-1);
    end
    delay_buffer(1) = y_undelayed;
   
    % 4. OUTPUT
    y = single(y_undelayed - y_delayed);
   
    % SAVE STATE
    y_undelayed_last = y_undelayed;
end

== matlab function c71_car0_template/Variant Display Maneuver/DisplayManeuver ==
  data: carid input; man input
function displayManuever(carid, man)
coder.extrinsic('line');

persistent config lineObj;

if isempty(config)
    config = mbc_config();
end

if isempty(lineObj)
    %figure(1);
    lineObj = line(man.points(2,1:man.breakslen), man.points(3,1:man.breakslen), 'Color', config.car.colors{carid+1}, 'LineStyle', '-');
end

set(lineObj, 'XData', man.points(2,1:man.breakslen), 'YData', man.points(3,1:man.breakslen));
end

== matlab function c71_car0_template/Motion Control and carinputs msg/Motion Control/pedalctrl/MATLAB Function2 ==
  data: u input; un output; P_p_vss_table parameter; P_p_un_table parameter; P_p_k parameter
function un = normalize_longitudinal_input(u, P_p_vss_table, P_p_un_table, P_p_k)

    ku = P_p_k;
    v_table = P_p_vss_table;
    un_table = P_p_un_table;
    % What steady-state speed would the nominal model
    % produce for this controller input?
    v_equiv = ku * u;

    % Find the real actuator input that produces
    % approximately the same steady-state speed
    un = interp1(v_table, un_table, ...
                 v_equiv, 'linear', 'extrap');

end

== matlab function c71_car0_template/Motion Control and carinputs msg/Motion Control/MATLAB Function ==
  data: spline input; states input; pedal output; delta output
function [pedal, delta] = MPC(spline, states)

    % states: [vr, s1, s2, psi] % until now I don't see why x is needed
    
    N = 20; % i wanted to use param but codegen does not support fmincon_option type
    
    coder.extrinsic('mpc_step_external');
    
    persistent u_warm
    
    if isempty(u_warm)
        u_warm = zeros(2*N,1);
    else
        % u_warm = [1 2 3 ... 99 100 101 102]
        % u_warm = [3 4 5 ... 101 102 101 102]
        u_warm(1:end-2) = u_warm(3:end); 
        % u_warm(end-1) = u_warm(end-3); % feel like unnecessary, is it?
        % u_warm(end)   = u_warm(end-2);
    end
    
    persistent u_last
    if isempty(u_last)
        u_last = zeros(2,1);
    end
    
    u_opt = zeros(2*N, 1); % this is necessary for codegen
    u_opt = mpc_step_external(states, u_warm, u_last, spline);
    u_warm = u_opt;
    u_last = [u_warm(1); u_warm(2)];
    
    pedal = single(u_opt(1));
    delta = single(u_opt(2));

end

== matlab function c71_car0_template/Motion Control and carinputs msg/Motion Control/pedalctrl/GP ==
  data: u input; y output; P_p_Tt parameter; P_dt parameter; P_p_T parameter; P_p_k parameter
function y = SmithPredictor(u, P_p_Tt, P_dt, P_p_T, P_p_k)
    % SMITH PREDICTOR IMPLEMENTATION
    % Calculates the difference between undelayed and delayed plant responses
   
    % delay_steps = round(P_p_Tt / P_dt);
   
    % if delay_steps < 1
    %     delay_steps = 1;
    % end

    delay_steps = 4;
   
    % MEMORY VARIABLES
    persistent y_undelayed_last
    persistent delay_buffer
   
    % INITIALIZATION
    if isempty(y_undelayed_last)
        y_undelayed_last = single(0);
        delay_buffer = zeros(delay_steps, 1, 'single');
    end
   
    % DYNAMIC BUFFER RESIZING
    if length(delay_buffer) ~= delay_steps
        new_buffer = zeros(delay_steps, 1, 'single');
        elements_to_copy = min(length(delay_buffer), delay_steps);
        new_buffer(1:elements_to_copy) = delay_buffer(1:elements_to_copy);
        delay_buffer = new_buffer;
    end
   
    % 1. UNDELAYED PLANT MODEL (Forward Euler)
    y_undelayed = y_undelayed_last + single(P_dt / P_p_T) * (single(P_p_k) * u - y_undelayed_last);
    % can try the exact
   
    % 2. DELAYED PLANT MODEL
    y_delayed = delay_buffer(end);
   
    % 3. BUFFER UPDATE
    if length(delay_buffer) > 1
        delay_buffer(2:end) = delay_buffer(1:end-1);
    end
    delay_buffer(1) = y_undelayed;
   
    % 4. OUTPUT
    y = single(y_undelayed - y_delayed);
   
    % SAVE STATE
    y_undelayed_last = y_undelayed;
end

== matlab function c71_car0_template/Receive maneuver/ROS2/MATLAB Function ==
  data: isnew input; rosmsg input; msg output Bus: DRIVEMANEUVER; P_max_breakslen parameter uint32; cpseq input
function msg = ros2msg(isnew, rosmsg, P_max_breakslen, cpseq)
msg = struct( ...
    'vmax', rosmsg.vmax, ...
    'type', rosmsg.type, ...
    'xref', rosmsg.xref, ...
    'lapCount', rosmsg.lapcount, ...
    'disableLaneMonitor', false, ...
    'isnew', isnew, ...
    'breakslen', rosmsg.breaks_SL_Info.CurrentLength, ...
    'points', [ rosmsg.breaks' ; rosmsg.s1' ; rosmsg.s2' ], ...
    'coefs', zeros(P_max_breakslen*2, 4, 'single'), ...
    'segments', rosmsg.segments', ...
    'periodic', rosmsg.periodic, ...
    'cpseq', cpseq);
msg.coefs(1:2:end-1,:) = reshape(rosmsg.spline_coefs1, 4, P_max_breakslen)';
msg.coefs(2:2:end,:) = reshape(rosmsg.spline_coefs2, 4, P_max_breakslen)';
end

== matlab function c71_car0_template/Motion Control and carinputs msg/Motion Control/pedalctrl/G_R1 ==
  data: e input; u output; e_last input; ui_last input; ui output; P_p_un_max parameter
function [u, ui] = pi_controller(e,e_last,ui_last,P_p_un_max)
   kr=0.177;
   Ti=0.12;
   ki=kr/Ti;
   T_sampling=0.025;
   
   up = kr*e;
   ui_increment = (T_sampling/2)*ki*(e+e_last);
   u_test = up + ui_last + ui_increment;

   if abs(u_test) > P_p_un_max
       u = P_p_un_max * sign(u_test);
       ui = double(ui_last);
   else
       u = u_test;
       ui = double(ui_last + ui_increment);
   end

   % u = single(u);
end

== matlab function c71_car0_template/Motion Control and carinputs msg/Motion Control/steeringctrl/MATLAB Function ==
  data: vr input; delta output
function delta = feedback_test_fcn(vr)

if(vr<10)
    delta = -0.9;
else
    delta = -0.85;
end

end

== matlab function c71_car0_template/Motion Control and carinputs msg/Motion Control/pedalctrl/MATLAB Function ==
  data: vr input; pedal output
function pedal = feedback_test_fcn(vr)

if(vr<10)
    pedal = 0.1;
else
    pedal = 0.0;
end

end

== matlab function c71_car0_template/Motion Control and carinputs msg/Motion Control/steeringctrl/MATLAB Function1 ==
  data: spline input; v_ref input; kappa_star output; s input; psi input; v_star output; s_star output; psi_star output; P_p_Tt parameter; s output; psi output
function [kappa_star, v_star, s_star,psi_star, s, psi]   = Reference_pf(spline,v_ref,s,psi, P_p_Tt)
    % decompose bus
    breakslen=spline.breakslen;
    points=spline.points;
    coefs=spline.coefs;
    periodic=spline.periodic;
    
    % get reference (closest points on trajectory)
    [w,~]=mbc_spline_get_reference(s,breakslen,points,coefs,periodic,...
        v_ref,P_p_Tt);
    psi_star=w(2);
    s_star=[w(3);w(4)];
    kappa_star=w(5);
    v_star=v_ref; %v* is needed for lookahead due to deadtime

end

== matlab function c71_car0_template/Motion Control and carinputs msg/Motion Control/steeringctrl/MATLAB Function2 ==
  data: kappa_star input; delta_star output; P_p_l parameter
function delta_star = ff_pf(kappa_star, P_p_l)
    delta_star=atan(P_p_l*kappa_star);
end

== matlab function c71_car0_template/Motion Control and carinputs msg/Motion Control/steeringctrl/MATLAB Function3 ==
  data: v_star input; delta_e output; s_star input; psi_star input; s input; psi input; P_p_l parameter; P_p_Tsteer parameter
function delta_e = fb_pf(v_star, s_star,psi_star,s,psi,P_p_l, P_p_Tsteer)
    %control deviation (see slideset 9 slide 13)
    sc2e=(s(2)-s_star(2))*cos(psi_star)-(s(1)-s_star(1))*sin(psi_star);
    % psi_e = psi - psi_star;
    % if abs(psi_e) < pi
    %     psi_e = -
    psi_e = atan2(sin(psi - psi_star), cos(psi - psi_star)); % wrapped psi_e=psi-psi_star
    
    % Tw=0.175; %[s] time constant of pt1 dynamics

    %control law (see slideset 9 slide 20)
    % delta_e = -P_p_l*sc2e/(Tw^2 * v_star^2) - 2*P_p_l*psi_e/(Tw*v_star);

    v_min = 0.05;  % TODO: minimum effective speed, tune this
    v_eff = max(abs(v_star), v_min);

    delta_e = -P_p_l*sc2e/(P_p_Tsteer^2 * v_eff^2) ...
        -2*P_p_l*psi_e/(P_p_Tsteer*v_eff);

== matlab function c71_car0_template/Motion Control and carinputs msg/Motion Control/steeringctrl/receding horizon LQR ==
  data: spline input; vr input; delta output; s input; psi input; params_lqr parameter
function delta = deviationLQR(spline, vr, s, psi, params_lqr)

N  = 10;
Ta = params_lqr.Ta;
l  = params_lqr.l;

%% Current linearization velocity

v_min = 0.03;
v_lin = max(abs(vr), v_min);

%% Build fresh reference preview

refs = lqr_build_reference(s, vr, spline, params_lqr);

%% Build LTV system

A = zeros(3,3,N);
B = zeros(3,1,N);

for i = 1:N

    psi_ref   = refs.psi(i);
    delta_ref = refs.delta(i);

    A(:,:,i) = ...
        [1 0 -Ta*v_lin*sin(psi_ref);
         0 1  Ta*v_lin*cos(psi_ref);
         0 0  1];

    B(:,:,i) = ...
        [0;
         0;
         Ta*v_lin/(l*cos(delta_ref)^2)];
end

sys.A = A;
sys.B = B;

%% DP backward recursion

[K_matrix, ~] = dp_backward_recursion( ...
    sys, params_lqr.weights, N);

%% Current deviation

e_psi = atan2( ...
    sin(psi - refs.psi(1)), ...
    cos(psi - refs.psi(1)));

dx = [s(1) - refs.s(1,1);
      s(2) - refs.s(2,1);
      e_psi];

%% Use only first gain

delta_fb = K_matrix(:,:,1) * dx;

%% Feedforward + feedback

delta = refs.delta(1) + delta_fb;

end

== matlab function c71_car0_template/Motion Control and carinputs msg/Motion Control/steeringctrl/augmentedLQR ==
  data: spline input; delta output; s input; psi input; vr input; upast input; upast_new output; params_lqr parameter
function [delta, upast_new] = deviationLQR( ...
    spline, s, psi, vr, upast, params_lqr)

%% ================================================================
% Parameters
% ================================================================

N  = 20;
Ta = params_lqr.Ta;
l  = params_lqr.l;

% Input delay
d = 4;          % 100 ms / 25 ms
nx = 2;
naug = nx + d;

%% ================================================================
% Velocity used for prediction / linearization
% ================================================================

v_min = 0.03;
v_lin = max(abs(vr), v_min);

%% ================================================================
% Fresh reference preview
% ================================================================

refs = lqr_build_reference(s, v_lin, spline, params_lqr);

%% ================================================================
% Build 2-state LTV model
%
% x_e = [sc2e;
%        psi_e]
%
% u_e = delta - delta_ref
% ================================================================

A = zeros(2,2,N);
B = zeros(2,1,N);

for i = 1:N

    % Use reference speed over prediction horizon
    v_k = refs.v(i);

    % Protect against very low speed
    v_k = max(abs(v_k), v_min);

    delta_k = refs.delta(i);

    b = v_k / (l*cos(delta_k)^2);

    % Exact ZOH discretization
    A(:,:,i) = ...
        [1, Ta*v_k;
         0, 1];

    B(:,:,i) = ...
        [0.5*Ta^2*v_k*b;
         Ta*b];

end

%% ================================================================
% Augment system with d-step input delay
%
% z_k =
%
% [ x_e,k     ]
% [ u_e,k-1   ]
% [ u_e,k-2   ]
% [ ...       ]
% [ u_e,k-d   ]
%
% The plant receives u_e,k-d.
% ================================================================

Aaug = zeros(naug,naug,N);
Baug = zeros(naug,1,N);

for k = 1:N

    Ak = A(:,:,k);
    Bk = B(:,:,k);

    %% Physical state dynamics
    %
    % x_{k+1} = Ak*x_k + Bk*u_{k-d}

    Aaug(1:nx,1:nx,k) = Ak;

    % Last delay state = u_{k-d}
    Aaug(1:nx,nx+d,k) = Bk;

    %% New command enters delay chain
    %
    % q1(k+1) = u(k)

    Baug(nx+1,1,k) = 1;

    %% Shift delay states
    %
    % q2(k+1) = q1(k)
    % q3(k+1) = q2(k)
    % ...

    for j = 2:d
        Aaug(nx+j,nx+j-1,k) = 1;
    end

end

sys_aug.A = Aaug;
sys_aug.B = Baug;

%% ================================================================
% Augmented cost
% ================================================================

weights_aug.Q = blkdiag( ...
    params_lqr.weights.Q, ...
    zeros(d));

weights_aug.P = blkdiag( ...
    params_lqr.weights.P, ...
    zeros(d));

weights_aug.R = params_lqr.weights.R;

%% ================================================================
% DP backward recursion
% ================================================================

[K_aug, ~] = dp_backward_recursion( ...
    sys_aug, ...
    weights_aug, ...
    N);

%% ================================================================
% Current deviation state
% ================================================================

psi_ref = refs.psi(1);

e_psi = atan2( ...
    sin(psi - psi_ref), ...
    cos(psi - psi_ref));

% Cross-track error expressed in reference frame
sc2e = ...
    (s(2) - refs.s(2,1))*cos(psi_ref) ...
  - (s(1) - refs.s(1,1))*sin(psi_ref);

xe = [sc2e;
      e_psi];

%% ================================================================
% Augmented feedback state
%
% upast must be 4x1:
%
% [u_e,k-1;
%  u_e,k-2;
%  u_e,k-3;
%  u_e,k-4]
% ================================================================

z = [xe;
     upast];

%% ================================================================
% Use first receding-horizon gain
% ================================================================

K0 = K_aug(:,:,1);

delta_fb = K0*z;

%% ================================================================
% Actual steering command
% ================================================================

delta_ref = refs.delta(1);

delta = delta_ref + delta_fb;

%% Steering saturation

delta_max = 0.93;

delta = min(max(delta, -delta_max), delta_max);

%% ================================================================
% Update delay history
%
% Store DEVIATION steering, not total steering.
%
% new history:
%
% [u_e,k;
%  u_e,k-1;
%  u_e,k-2;
%  u_e,k-3]
% ================================================================

upast_new = double([delta_fb;
             upast(1:d-1)]);

end
